simulink model "autopilot_stateflow_sldv_P05_test"  (Simulink 8.8)
settings: Solver=FixedStepDiscrete  StartTime=0.0  StopTime=10.0  FixedStep=0.1  RelTol=1e-3  EnableMultiTasking=on
libraries: simulink x38, sldvlib x17
settings OptimizationCC: ExpressionDepthLimit=2147483647
settings DebuggingCC: SolverPrmCheckMsg=warning
settings GRTTargetCC: CombineOutputUpdateFcns=on  GRTInterface=off
settings ConfigComp: DVMode=PropertyProving  DVMaxProcessTime=30000  DVTestSuiteOptimization=CombinedObjectives (Nonlinear Extended)  DVDetectDeadLogic=on  DVDetectActiveLogic=on  DVDetectFloatOverflow=off  DVProvingStrategy=FindViolation

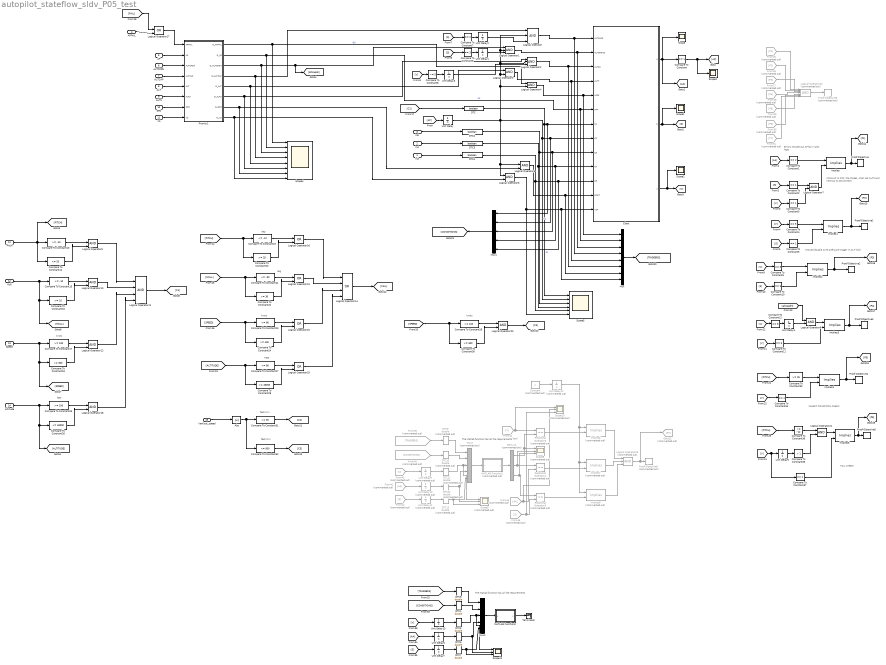
== system autopilot_stateflow_sldv_P05_test ==
  note: The Matlab function has all the requirements
  note: While AP is OFF, the Modes, shall set ALTS and
      | Vertical to Disconnect
  note: feet/min
  note: knots
  note: feet
  note: knots
  note: deg
  note: deg
  note: knots
  note: Feet
  note: feet/min
  note: FAIL CHECK
  note: INHIBIT CONDITION CHECK
  note: Missed disable ALTS software trigger in ALT hold
  note: Errors
      | Missed out AP fail in alts logic
  note: The Matlab function has all the requirements
  In3 : Inport
  In4 : Inport  Port=2
  In5 : Inport  Port=3
  APFAIL : Inport  Port=4
  AP : Inport  Port=5
  ALTCPDN : Inport  Port=6
  ALTCAP : Inport  Port=7
  ALT : Inport  Port=8
  ALTS : Inport  Port=9
  SPD : Inport  Port=10
  VS : Inport  Port=11
  Pitch : Inport  Port=12
  Speed : Inport  Port=13
  Altitude : Inport  Port=14
  Vertical_speed : Inport  Port=15
  Abs : Abs
  Chart : Stateflow chart  TreatAsAtomicUnit=on
  Compare To Constant{,2..3,5,34,37} (6 alike) : simulink/Logic and Bit Operations/Compare To Constant  relop===  const=1  OutDataTypeStr=boolean
  Compare To Constant1 : simulink/Logic and Bit Operations/Compare To Constant  relop===  const=2  OutDataTypeStr=boolean
  Compare To Constant10 : simulink/Logic and Bit Operations/Compare To Constant  relop===  const=3  OutDataTypeStr=boolean
  Compare To Constant11 : simulink/Logic and Bit Operations/Compare To Constant  relop===  const=5  OutDataTypeStr=boolean
  Compare To Constant12 : simulink/Logic and Bit Operations/Compare To Constant  relop===  const=6  OutDataTypeStr=boolean
  Compare To Constant13 : simulink/Logic and Bit Operations/Compare To Constant  relop=>=  const=-10  OutDataTypeStr=boolean
  Compare To Constant14 : simulink/Logic and Bit Operations/Compare To Constant  relop=<=  const=20  OutDataTypeStr=boolean
  Compare To Constant15 : simulink/Logic and Bit Operations/Compare To Constant  relop=>=  const=-10  OutDataTypeStr=boolean
  Compare To Constant16 : simulink/Logic and Bit Operations/Compare To Constant  relop=<=  const=10  OutDataTypeStr=boolean
  Compare To Constant17 : simulink/Logic and Bit Operations/Compare To Constant  relop=>=  const=100  OutDataTypeStr=boolean
  Compare To Constant18 : simulink/Logic and Bit Operations/Compare To Constant  relop=<=  const=300  OutDataTypeStr=boolean
  Compare To Constant19 : simulink/Logic and Bit Operations/Compare To Constant  relop=<=  const=-12  OutDataTypeStr=boolean
  Compare To Constant20 : simulink/Logic and Bit Operations/Compare To Constant  relop=>=  const=25  OutDataTypeStr=boolean
  Compare To Constant21 : simulink/Logic and Bit Operations/Compare To Constant  relop=<=  const=-30  OutDataTypeStr=boolean
  Compare To Constant22 : simulink/Logic and Bit Operations/Compare To Constant  relop=>=  const=30  OutDataTypeStr=boolean
  Compare To Constant23 : simulink/Logic and Bit Operations/Compare To Constant  relop=<=  const=80  OutDataTypeStr=boolean
  Compare To Constant24 : simulink/Logic and Bit Operations/Compare To Constant  relop=>=  const=400  OutDataTypeStr=boolean
  Compare To Constant25 : simulink/Logic and Bit Operations/Compare To Constant  relop=>=  const=100  OutDataTypeStr=boolean
  Compare To Constant26 : simulink/Logic and Bit Operations/Compare To Constant  relop=<=  const=40000  OutDataTypeStr=boolean
  Compare To Constant27 : simulink/Logic and Bit Operations/Compare To Constant  relop=<=  const=80  OutDataTypeStr=boolean
  Compare To Constant28 : simulink/Logic and Bit Operations/Compare To Constant  relop=>=  const=45000  OutDataTypeStr=boolean
  Compare To Constant29 : simulink/Logic and Bit Operations/Compare To Constant  relop=>=  const=120  OutDataTypeStr=boolean
  Compare To Constant30 : simulink/Logic and Bit Operations/Compare To Constant  relop=<=  const=300  OutDataTypeStr=boolean
  Compare To Constant31 : simulink/Logic and Bit Operations/Compare To Constant  relop=>=  const=50  OutDataTypeStr=boolean
  Compare To Constant32 : simulink/Logic and Bit Operations/Compare To Constant  relop=<=  const=500  OutDataTypeStr=boolean
  Compare To Constant33 : simulink/Logic and Bit Operations/Compare To Constant  relop=>=  const=25  OutDataTypeStr=boolean
  Compare To Constant35 : simulink/Logic and Bit Operations/Compare To Constant  relop=>  const=1  OutDataTypeStr=boolean
  Compare To Constant36 : simulink/Logic and Bit Operations/Compare To Constant  relop=<=  const=-12  OutDataTypeStr=boolean
  Compare To Constant4 : simulink/Logic and Bit Operations/Compare To Constant  relop===  const=5  OutDataTypeStr=boolean
  Compare To Constant6 : simulink/Logic and Bit Operations/Compare To Constant  relop===  const=3  OutDataTypeStr=boolean
  Compare To Constant7 : simulink/Logic and Bit Operations/Compare To Constant  relop===  const=2  OutDataTypeStr=boolean
  Compare To Constant8 : simulink/Logic and Bit Operations/Compare To Constant  relop=~=  const=5  OutDataTypeStr=boolean
  Compare To Constant9 : simulink/Logic and Bit Operations/Compare To Constant  relop===  const=6  OutDataTypeStr=boolean
  Constant : Constant  Commented=on
  DTC{,2..4} (4 alike) : DataTypeConversion  OutDataTypeStr=boolean
  DTC{1,5..8} (5 alike) : DataTypeConversion  OutDataTypeStr=double
  DTC{9..13} (5 alike) : DataTypeConversion  Commented=on  OutDataTypeStr=double
  Demux1 : Demux  Commented=on  Outputs=3
  From25 : From  Commented=on  GotoTag=P1
  From26 : From  Commented=on  GotoTag=P2
  From27 : From  Commented=on  GotoTag=P3
  From28 : From  Commented=on  GotoTag=P4
  From29 : From  Commented=on  GotoTag=P5
  From30 : From  Commented=on  GotoTag=P6
  From31 : From  Commented=on  GotoTag=P7
  From39 : From  Commented=on  GotoTag=TRIGGERS
  From40 : From  Commented=on  GotoTag=CONDITIONS
  From41 : From  Commented=on  GotoTag=AA
  From42 : From  Commented=on  GotoTag=S
  From43 : From  Commented=on  GotoTag=V
  From44 : From  Commented=on  GotoTag=V
  From45 : From  Commented=on  GotoTag=AA
  From46 : From  Commented=on  GotoTag=S
  Goto22 : Goto  Commented=on  GotoTag=P7
  Implies{,1..5} (6 alike) : sldvlib/Verification Utilities/Implies
  Implies6 : sldvlib/Verification Utilities/Implies  Commented=on
  Implies7 : sldvlib/Verification Utilities/Implies  Commented=on
  Implies8 : sldvlib/Verification Utilities/Implies  Commented=on
  Logical Operator : Logic  Inputs=3  IconShape=distinctive  AllPortsSameDT=off  OutDataTypeStr=boolean
  Logical Operator1 : Logic  Inputs=3  IconShape=distinctive  AllPortsSameDT=off  OutDataTypeStr=boolean
  Logical Operator{3..6,9..10,12,18,20} (9 alike) : Logic  IconShape=distinctive  AllPortsSameDT=off  OutDataTypeStr=boolean
  Logical Operator11 : Logic  Inputs=4  IconShape=distinctive  AllPortsSameDT=off  OutDataTypeStr=boolean
  Logical Operator{13,15..17,19} (5 alike) : Logic  Operator=OR  IconShape=distinctive  AllPortsSameDT=off  OutDataTypeStr=boolean
  Logical Operator14 : Logic  Operator=OR  Inputs=4  IconShape=distinctive  AllPortsSameDT=off  OutDataTypeStr=boolean
  Logical Operator2 : Logic  Inputs=3  IconShape=distinctive  AllPortsSameDT=off  OutDataTypeStr=boolean
  Logical Operator21 : Logic  AllPortsSameDT=off  OutDataTypeStr=boolean
  Logical Operator22 : Logic  Commented=on  Inputs=7  IconShape=distinctive  AllPortsSameDT=off  OutDataTypeStr=boolean
  Logical Operator23 : Logic  Commented=on  Inputs=3  IconShape=distinctive  AllPortsSameDT=off  OutDataTypeStr=boolean
  Logical Operator7 : Logic  AllPortsSameDT=off  OutDataTypeStr=boolean
  Logical Operator8 : Logic  AllPortsSameDT=off  OutDataTypeStr=boolean
  MATLAB Function1 : MATLAB Function  Commented=on  TreatAsAtomicUnit=on
  MATLAB Function2 : MATLAB Function  TreatAsAtomicUnit=on
  Mux : Mux  Inputs=8
  Mux1 : Mux  Inputs=5
  Mux2 : Mux  Inputs=5
  Mux3 : Mux  Commented=on  Inputs=5
  Priority1 : Subsystem
  Proof Objective{,1..5} (6 alike) : sldvlib/Objectives and Constraints/Proof Objective  enabled=off  customAVTBlockType=Proof Objective  intervals=true  dispValues=on  outEnabled=off  enableStopSim=off
      settings: AttributesFormatString=%<intervals>
  Proof Objective6 : sldvlib/Objectives and Constraints/Proof Objective  Commented=on  enabled=on  customAVTBlockType=Proof Objective  intervals=true  dispValues=on  outEnabled=off  enableStopSim=off
      settings: AttributesFormatString=%<intervals>
  Proof Objective8 : sldvlib/Objectives and Constraints/Proof Objective  Commented=on  enabled=off  customAVTBlockType=Proof Objective  intervals=true  dispValues=on  outEnabled=off  enableStopSim=off
      settings: AttributesFormatString=%<intervals>
  Relational Operator3 : RelationalOperator  Commented=on  Operator===  OutDataTypeStr=boolean  RndMeth=Simplest
  Relational Operator4 : RelationalOperator  Commented=on  Operator===  OutDataTypeStr=boolean  RndMeth=Simplest
  Relational Operator5 : RelationalOperator  Commented=on  Operator===  OutDataTypeStr=boolean  RndMeth=Simplest
  Roll : InportShadow  Port=12
  Scope{,1..3} (4 alike) : Scope
  Scope10 : Scope  Commented=on  NumInputPorts=3
  Scope11 : Scope  NumInputPorts=3
  Scope4 : Scope  NumInputPorts=8
  Scope5 : Scope  NumInputPorts=6
  Scope8 : Scope  Commented=on  NumInputPorts=3
  Scope9 : Scope  Commented=on  NumInputPorts=3
  Terminator : Terminator
  Unit Delay{,1..5} (6 alike) : UnitDelay  SampleTime=-1
  Unit Delay10 : UnitDelay  Commented=on  InitialCondition=2  SampleTime=-1
  Unit Delay11 : UnitDelay  Commented=on  InitialCondition=1  SampleTime=-1
  Unit Delay12 : UnitDelay  Commented=on  SampleTime=-1
  Unit Delay13 : UnitDelay  InitialCondition=1  SampleTime=-1
  Unit Delay6 : UnitDelay  InitialCondition=2  SampleTime=-1
  Unit Delay7 : UnitDelay  InitialCondition=1  SampleTime=-1
  Unit Delay9 : UnitDelay  Commented=on  InitialCondition=1  SampleTime=-1
  wires:
  Priority1/2(O_AP) -> Mux/2, Chart/6(APT), Scope4/2  "ap"
  [C1] -> DTC/1
  In5/1 -> DTC2/1
  In4/1 -> DTC3/1
  In3/1 -> DTC4/1
  DTC/1 -> Scope5/1, Mux1/1, Chart/7(C1)  "C1"
  DTC2/1 -> Scope5/3, Mux1/3, Chart/9(C3)
  DTC3/1 -> Scope5/4, Mux1/4, Chart/10(C4)
  DTC4/1 -> Scope5/5, Mux1/5, Chart/11(C5)
  Compare To Constant/1 -> Scope3/1, [AP]
  Chart/1(A) -> [AA], Compare To Constant/1, Scope/1
  [AP] -> Unit Delay/1
  Chart/2(S) -> Scope1/1, [S]
  Chart/3(V) -> Scope2/1, [V]
  Unit Delay/1 -> Scope5/2, Mux1/2, Chart/8(C2), Logical Operator6/1, Logical Operator5/1, Logical Operator3/2, Logical Operator/2, Logical Operator1/2, Logical Operator2/2, Logical Operator4/2  "C2"
  Logical Operator/1 -> Mux/4, Chart/1(ALTCAPS)
  Priority1/4(O_ALTCAP) -> Logical Operator/1, Scope4/4
  Logical Operator1/1 -> Mux/3, Chart/2(ALTCPDNS)
  Priority1/3(O_ALTCPDN) -> [altcapdn], Logical Operator1/1, Scope4/3
  Logical Operator2/1 -> Mux/6, Chart/3(ALTSS)
  Priority1/6(O_ALTS) -> Logical Operator2/1, Scope4/6
  Logical Operator3/1 -> Mux/5, Chart/4(ALTT)
  Priority1/5(O_ALT) -> Logical Operator3/1, Scope4/5
  Logical Operator4/1 -> Mux/1, Chart/5(APFS)
  Priority1/1(O_APFAIL) -> Logical Operator4/1, Scope4/1  "fail"
  Priority1/7(O_SPD) -> Logical Operator5/2, Scope4/7
  Logical Operator5/1 -> Mux/7, Chart/12(SPDT)
  Logical Operator6/1 -> Scope5/6, Mux/8, Chart/13(VST)
  Priority1/8(O_VS) -> Logical Operator6/2, Scope4/8
  ALT/1 -> Priority1/5(ALT)
  AP/1 -> Priority1/2(AP)
  ALTCAP/1 -> Priority1/4(ALTCAP)
  ALTS/1 -> Priority1/6(ALTS)
  SPD/1 -> Priority1/7(SPD)
  VS/1 -> Priority1/8(VS)
  ALTCPDN/1 -> Priority1/3(ALTCPDN)
  Unit Delay1/1 -> Logical Operator1/3
  [S] -> Compare To Constant6/1
  Compare To Constant6/1 -> Unit Delay1/1
  [S] -> Compare To Constant7/1
  Compare To Constant7/1 -> Unit Delay2/1
  Unit Delay2/1 -> Logical Operator/3
  [V] -> Compare To Constant8/1
  Compare To Constant8/1 -> Unit Delay3/1
  Unit Delay3/1 -> Logical Operator2/3
  Pitch/1 -> [PITCH], Compare To Constant14/1, Compare To Constant13/1
  Compare To Constant13/1 -> Logical Operator9/1
  Compare To Constant14/1 -> Logical Operator9/2
  Roll/1 -> Compare To Constant15/1, [ROLL], Compare To Constant16/1
  Compare To Constant15/1 -> Logical Operator10/1
  Compare To Constant16/1 -> Logical Operator10/2
  Speed/1 -> [SPEED], Compare To Constant18/1, Compare To Constant17/1
  Compare To Constant17/1 -> Logical Operator12/1
  Compare To Constant18/1 -> Logical Operator12/2
  Logical Operator9/1 -> Logical Operator11/1
  Logical Operator10/1 -> Logical Operator11/2
  Logical Operator12/1 -> Logical Operator11/3
  Logical Operator11/1 -> [C1]
  [PITCH] -> Compare To Constant19/1, Compare To Constant20/1
  Compare To Constant19/1 -> Logical Operator16/1
  Compare To Constant20/1 -> Logical Operator16/2
  [ROLL] -> Compare To Constant22/1, Compare To Constant21/1
  Compare To Constant21/1 -> Logical Operator13/1
  Compare To Constant22/1 -> Logical Operator13/2
  [SPEED] -> Compare To Constant23/1, Compare To Constant24/1
  Compare To Constant23/1 -> Logical Operator15/1
  Compare To Constant24/1 -> Logical Operator15/2
  Logical Operator16/1 -> Logical Operator14/1
  Logical Operator13/1 -> Logical Operator14/2
  Logical Operator15/1 -> Logical Operator14/3
  Logical Operator14/1 -> [FAIL]
  APFAIL/1 -> Logical Operator17/2
  [FAIL] -> Logical Operator17/1
  Logical Operator17/1 -> Priority1/1(APFAIL)
  Altitude/1 -> Compare To Constant25/1, Compare To Constant26/1, [ALTITUDE]
  Compare To Constant25/1 -> Logical Operator18/1
  Compare To Constant26/1 -> Logical Operator18/2
  Logical Operator18/1 -> Logical Operator11/4
  [ALTITUDE] -> Compare To Constant28/1, Compare To Constant27/1
  Compare To Constant27/1 -> Logical Operator19/1
  Compare To Constant28/1 -> Logical Operator19/2
  Logical Operator19/1 -> Logical Operator14/4
  [SPEED] -> Compare To Constant30/1, Compare To Constant29/1
  Compare To Constant29/1 -> Logical Operator20/1
  Compare To Constant30/1 -> Logical Operator20/2
  Logical Operator20/1 -> [C3]
  Vertical_speed/1 -> Abs/1
  Abs/1 -> Compare To Constant32/1, Compare To Constant31/1
  Compare To Constant31/1 -> [C4]
  Compare To Constant32/1 -> [C5]
  Compare To Constant1/1 -> Implies/1
  [AA] -> Compare To Constant1/1
  [S] -> Compare To Constant2/1
  Compare To Constant2/1 -> Logical Operator7/1
  [V] -> Compare To Constant3/1
  Compare To Constant3/1 -> Logical Operator7/2
  Logical Operator7/1 -> Implies/2
  Implies/1 -> [P1], Proof Objective/1
  [V] -> Compare To Constant4/1
  Compare To Constant4/1 -> Implies1/1
  [S] -> Compare To Constant5/1
  Compare To Constant5/1 -> Implies1/2
  Implies1/1 -> [P2], Proof Objective1/1
  [V] -> Compare To Constant9/1
  Compare To Constant9/1 -> Implies2/1
  [S] -> Compare To Constant10/1
  Compare To Constant10/1 -> Implies2/2
  Implies2/1 -> [P3], Proof Objective2/1
  [V] -> Compare To Constant12/1
  Compare To Constant12/1 -> Unit Delay4/1
  [V] -> Compare To Constant11/1
  Implies3/1 -> [P4], Proof Objective3/1
  Unit Delay4/1 -> Logical Operator8/2
  Logical Operator8/1 -> Implies3/1
  [altcapdn] -> Logical Operator8/1
  Compare To Constant11/1 -> Implies3/2
  [PITCH] -> Compare To Constant33/1
  Compare To Constant33/1 -> Implies4/1
  [V] -> Compare To Constant34/1
  Compare To Constant34/1 -> Implies4/2
  Implies4/1 -> [P5], Proof Objective4/1
  [V] -> Compare To Constant37/1, Unit Delay5/1
  [PITCH] -> Compare To Constant36/1
  Unit Delay5/1 -> Compare To Constant35/1
  Compare To Constant35/1 -> Logical Operator21/2
  Compare To Constant36/1 -> Logical Operator21/1
  Logical Operator21/1 -> Implies5/1
  Compare To Constant37/1 -> Implies5/2
  Implies5/1 -> [P6], Proof Objective5/1
  From28/1 -> Logical Operator22/4
  From27/1 -> Logical Operator22/3
  From29/1 -> Logical Operator22/5
  From26/1 -> Logical Operator22/2
  From30/1 -> Logical Operator22/6
  From25/1 -> Logical Operator22/1
  Logical Operator22/1 -> Proof Objective6/1
  Mux/1 -> [TRIGGERS]
  Mux1/1 -> [CONDITIONS]
  From40/1 -> DTC10/1
  From39/1 -> DTC9/1
  From43/1 -> Unit Delay9/1
  From41/1 -> Unit Delay10/1
  From42/1 -> Unit Delay11/1
  Mux3/1 -> MATLAB Function1/1(u)
  Unit Delay9/1 -> DTC11/1
  Unit Delay10/1 -> DTC12/1
  Unit Delay11/1 -> DTC13/1
  MATLAB Function1/1(y) -> Demux1/1
  From44/1 -> Scope10/1, Relational Operator3/1
  Demux1/1 -> Relational Operator3/2, Scope8/1
  Demux1/2 -> Relational Operator4/1, Scope8/2
  From45/1 -> Scope10/2, Relational Operator4/2
  Demux1/3 -> Relational Operator5/1, Scope8/3
  From46/1 -> Scope10/3, Relational Operator5/2
  DTC9/1 -> Mux3/1
  DTC10/1 -> Mux3/2
  DTC11/1 -> Mux3/3, Scope9/1
  DTC12/1 -> Mux3/4, Scope9/2
  DTC13/1 -> Mux3/5, Scope9/3
  Relational Operator3/1 -> Implies6/2
  Unit Delay12/1 -> Implies8/1, Implies7/1, Implies6/1
  Constant/1 -> Unit Delay12/1
  Relational Operator4/1 -> Implies7/2
  Relational Operator5/1 -> Implies8/2
  Implies7/1 -> Logical Operator23/2
  Implies6/1 -> Logical Operator23/1
  Implies8/1 -> Logical Operator23/3
  Logical Operator23/1 -> Goto22/1, Proof Objective8/1
  From31/1 -> Logical Operator22/7
  [CONDITIONS] -> DTC1/1
  [TRIGGERS] -> DTC8/1
  [V] -> Unit Delay13/1
  [AA] -> Unit Delay6/1
  [S] -> Unit Delay7/1
  Mux2/1 -> MATLAB Function2/1(u)
  Unit Delay13/1 -> DTC5/1
  Unit Delay6/1 -> DTC6/1
  Unit Delay7/1 -> DTC7/1
  DTC8/1 -> Mux2/1
  DTC1/1 -> Mux2/2
  DTC5/1 -> Scope11/1, Mux2/3
  DTC6/1 -> Scope11/2, Mux2/4
  DTC7/1 -> Scope11/3, Mux2/5
  MATLAB Function2/1(y) -> Terminator/1

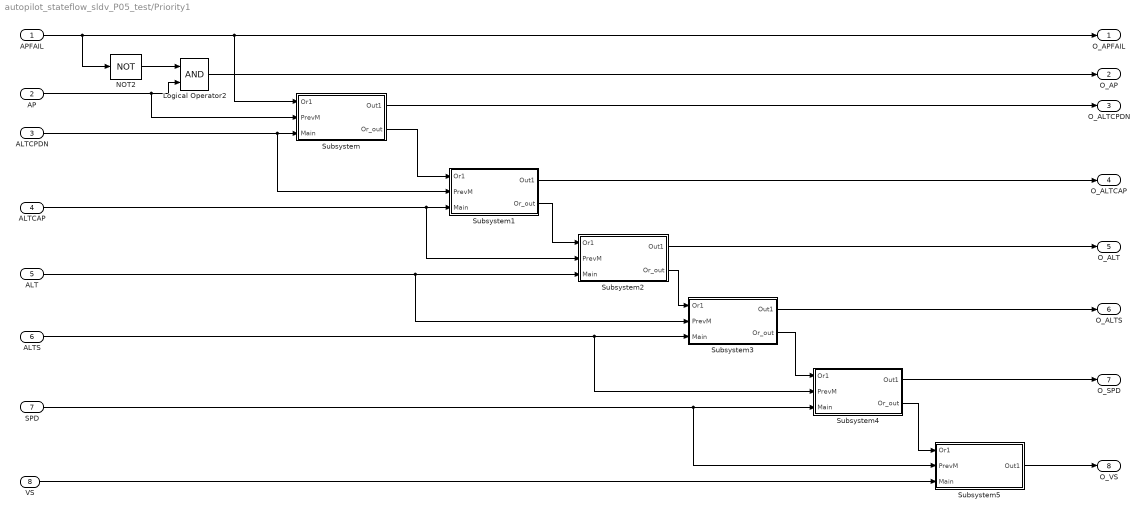
== system autopilot_stateflow_sldv_P05_test/Priority1 ==
  APFAIL : Inport
  AP : Inport  Port=2
  ALTCPDN : Inport  Port=3
  ALTCAP : Inport  Port=4
  ALT : Inport  Port=5
  ALTS : Inport  Port=6
  SPD : Inport  Port=7
  VS : Inport  Port=8
  Logical Operator2 : Logic  AllPortsSameDT=off  OutDataTypeStr=boolean
  NOT2 : Logic  Operator=NOT  AllPortsSameDT=off  OutDataTypeStr=boolean
  Subsystem : Subsystem
  Subsystem1 : Subsystem
  Subsystem2 : Subsystem
  Subsystem3 : Subsystem
  Subsystem4 : Subsystem
  Subsystem5 : Subsystem
  O_APFAIL : Outport
  O_AP : Outport  Port=2
  O_ALTCPDN : Outport  Port=3
  O_ALTCAP : Outport  Port=4
  O_ALT : Outport  Port=5
  O_ALTS : Outport  Port=6
  O_SPD : Outport  Port=7
  O_VS : Outport  Port=8
  wires:
  AP/1 -> Subsystem/2(PrevM), Logical Operator2/2
  APFAIL/1 -> Subsystem/1(Or1), O_APFAIL/1, NOT2/1
  NOT2/1 -> Logical Operator2/1
  Logical Operator2/1 -> O_AP/1
  ALTCPDN/1 -> Subsystem1/2(PrevM), Subsystem/3(Main)
  Subsystem/2(Or_out) -> Subsystem1/1(Or1)
  ALTCAP/1 -> Subsystem2/2(PrevM), Subsystem1/3(Main)
  Subsystem/1(Out1) -> O_ALTCPDN/1
  Subsystem1/1(Out1) -> O_ALTCAP/1
  Subsystem1/2(Or_out) -> Subsystem2/1(Or1)
  ALT/1 -> Subsystem3/2(PrevM), Subsystem2/3(Main)
  Subsystem2/1(Out1) -> O_ALT/1
  Subsystem2/2(Or_out) -> Subsystem3/1(Or1)
  ALTS/1 -> Subsystem4/2(PrevM), Subsystem3/3(Main)
  Subsystem3/1(Out1) -> O_ALTS/1
  Subsystem3/2(Or_out) -> Subsystem4/1(Or1)
  SPD/1 -> Subsystem5/2(PrevM), Subsystem4/3(Main)
  Subsystem4/1(Out1) -> O_SPD/1
  Subsystem4/2(Or_out) -> Subsystem5/1(Or1)
  VS/1 -> Subsystem5/3(Main)
  Subsystem5/1(Out1) -> O_VS/1

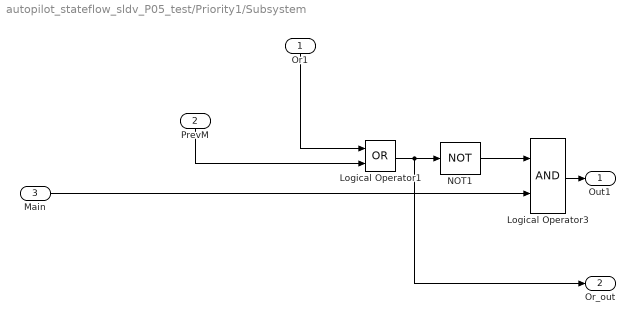
== system autopilot_stateflow_sldv_P05_test/Priority1/Subsystem ==
  Or1 : Inport
  PrevM : Inport  Port=2
  Main : Inport  Port=3
  Logical Operator1 : Logic  Operator=OR  AllPortsSameDT=off  OutDataTypeStr=boolean
  Logical Operator3 : Logic  AllPortsSameDT=off  OutDataTypeStr=boolean
  NOT1 : Logic  Operator=NOT  AllPortsSameDT=off  OutDataTypeStr=boolean
  Out1 : Outport
  Or_out : Outport  Port=2
  wires:
  Main/1 -> Logical Operator3/2
  Logical Operator1/1 -> Or_out/1, NOT1/1
  NOT1/1 -> Logical Operator3/1
  Or1/1 -> Logical Operator1/1
  Logical Operator3/1 -> Out1/1
  PrevM/1 -> Logical Operator1/2

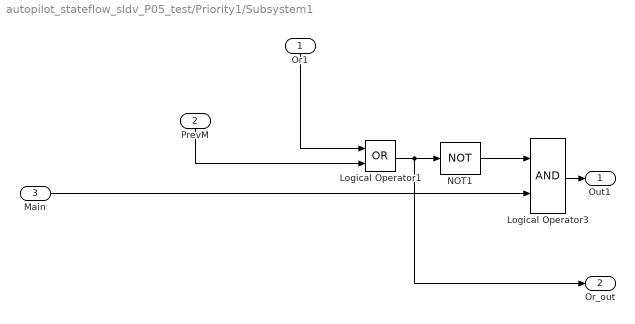
== system autopilot_stateflow_sldv_P05_test/Priority1/Subsystem1 ==
  Or1 : Inport
  PrevM : Inport  Port=2
  Main : Inport  Port=3
  Logical Operator1 : Logic  Operator=OR  AllPortsSameDT=off  OutDataTypeStr=boolean
  Logical Operator3 : Logic  AllPortsSameDT=off  OutDataTypeStr=boolean
  NOT1 : Logic  Operator=NOT  AllPortsSameDT=off  OutDataTypeStr=boolean
  Out1 : Outport
  Or_out : Outport  Port=2
  wires:
  PrevM/1 -> Logical Operator1/2
  Logical Operator3/1 -> Out1/1
  Or1/1 -> Logical Operator1/1
  NOT1/1 -> Logical Operator3/1
  Logical Operator1/1 -> NOT1/1, Or_out/1
  Main/1 -> Logical Operator3/2

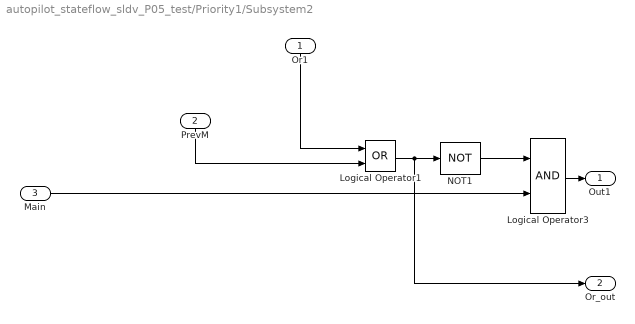
== system autopilot_stateflow_sldv_P05_test/Priority1/Subsystem2 ==
  Or1 : Inport
  PrevM : Inport  Port=2
  Main : Inport  Port=3
  Logical Operator1 : Logic  Operator=OR  AllPortsSameDT=off  OutDataTypeStr=boolean
  Logical Operator3 : Logic  AllPortsSameDT=off  OutDataTypeStr=boolean
  NOT1 : Logic  Operator=NOT  AllPortsSameDT=off  OutDataTypeStr=boolean
  Out1 : Outport
  Or_out : Outport  Port=2
  wires:
  Main/1 -> Logical Operator3/2
  Logical Operator1/1 -> Or_out/1, NOT1/1
  NOT1/1 -> Logical Operator3/1
  Or1/1 -> Logical Operator1/1
  Logical Operator3/1 -> Out1/1
  PrevM/1 -> Logical Operator1/2

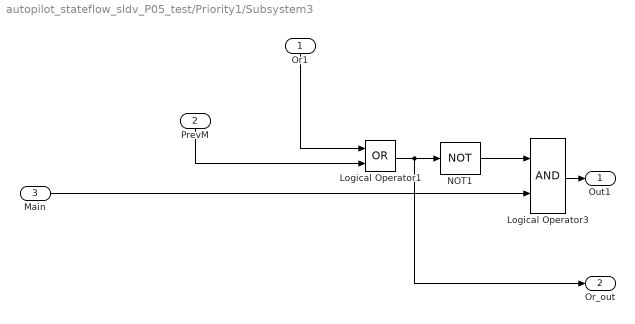
== system autopilot_stateflow_sldv_P05_test/Priority1/Subsystem3 ==
  Or1 : Inport
  PrevM : Inport  Port=2
  Main : Inport  Port=3
  Logical Operator1 : Logic  Operator=OR  AllPortsSameDT=off  OutDataTypeStr=boolean
  Logical Operator3 : Logic  AllPortsSameDT=off  OutDataTypeStr=boolean
  NOT1 : Logic  Operator=NOT  AllPortsSameDT=off  OutDataTypeStr=boolean
  Out1 : Outport
  Or_out : Outport  Port=2
  wires:
  PrevM/1 -> Logical Operator1/2
  Logical Operator3/1 -> Out1/1
  Or1/1 -> Logical Operator1/1
  NOT1/1 -> Logical Operator3/1
  Logical Operator1/1 -> NOT1/1, Or_out/1
  Main/1 -> Logical Operator3/2

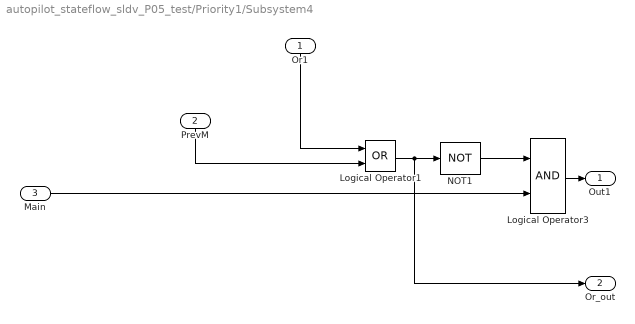
== system autopilot_stateflow_sldv_P05_test/Priority1/Subsystem4 ==
  Or1 : Inport
  PrevM : Inport  Port=2
  Main : Inport  Port=3
  Logical Operator1 : Logic  Operator=OR  AllPortsSameDT=off  OutDataTypeStr=boolean
  Logical Operator3 : Logic  AllPortsSameDT=off  OutDataTypeStr=boolean
  NOT1 : Logic  Operator=NOT  AllPortsSameDT=off  OutDataTypeStr=boolean
  Out1 : Outport
  Or_out : Outport  Port=2
  wires:
  Main/1 -> Logical Operator3/2
  Logical Operator1/1 -> Or_out/1, NOT1/1
  NOT1/1 -> Logical Operator3/1
  Or1/1 -> Logical Operator1/1
  Logical Operator3/1 -> Out1/1
  PrevM/1 -> Logical Operator1/2

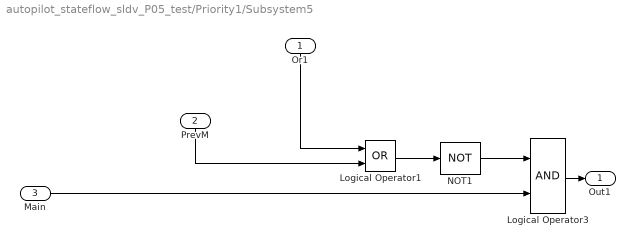
== system autopilot_stateflow_sldv_P05_test/Priority1/Subsystem5 ==
  Or1 : Inport
  PrevM : Inport  Port=2
  Main : Inport  Port=3
  Logical Operator1 : Logic  Operator=OR  AllPortsSameDT=off  OutDataTypeStr=boolean
  Logical Operator3 : Logic  AllPortsSameDT=off  OutDataTypeStr=boolean
  NOT1 : Logic  Operator=NOT  AllPortsSameDT=off  OutDataTypeStr=boolean
  Out1 : Outport
  wires:
  PrevM/1 -> Logical Operator1/2
  Logical Operator3/1 -> Out1/1
  Or1/1 -> Logical Operator1/1
  NOT1/1 -> Logical Operator3/1
  Logical Operator1/1 -> NOT1/1
  Main/1 -> Logical Operator3/2

== stateflow chart Chart ==
  state VERT [parallel]
    settings: executionOrder=1
    state DIS_01
      en: V = 1;
    state SPDH_03
      en: V = 3;
    state ALT_05
      en: V = 5;
    state PAH_02
      en: V = 2;
    state VS_04
      en: V = 4;
    state ALTSCAP_06
      en: V = 6;
    SPDH_03 -> DIS_01 [order 6] : [APFS & C2]
    (default) -> DIS_01
    SPDH_03 -> DIS_01 [order 1] : [APT & C2]
    SPDH_03 -> ALT_05 [order 4] : [ALTT & C5]
    DIS_01 -> PAH_02 : [APT & C1]
    PAH_02 -> SPDH_03 [order 2] : [SPDT & C3]
    ALT_05 -> DIS_01 [order 5] : [APFS & C2]
    ALT_05 -> SPDH_03 [order 2] : [SPDT & C3]
    ALT_05 -> DIS_01 [order 1] : [APT & C2]
    SPDH_03 -> PAH_02 [order 2] : [SPDT]
    VS_04 -> SPDH_03 [order 2] : [SPDT & C3]
    PAH_02 -> DIS_01 [order 6] : [APFS & C2]
    PAH_02 -> DIS_01 [order 1] : [APT & C2]
    ALTSCAP_06 -> DIS_01 [order 4] : [APFS & C2]
    ALTSCAP_06 -> DIS_01 [order 1] : [APT & C2]
    VS_04 -> DIS_01 [order 6] : [APFS & C2]
    VS_04 -> DIS_01 [order 1] : [APT & C2]
    SPDH_03 -> ALTSCAP_06 [order 5] : [ALTCAPS]
    SPDH_03 -> VS_04 [order 3] : [VST & C4]
    VS_04 -> ALT_05 [order 4] : [ALTT & C5]
    ALT_05 -> PAH_02 [order 4] : [ALTT]
    PAH_02 -> ALT_05 [order 4] : [ALTT & C5]
    ALTSCAP_06 -> ALT_05 [order 2] : [ALTT & C5]
    ALTSCAP_06 -> ALT_05 [order 3] : [ALTCPDNS]
    ALT_05 -> VS_04 [order 3] : [VST & C4]
    PAH_02 -> ALTSCAP_06 [order 5] : [ALTCAPS]
    PAH_02 -> VS_04 [order 3] : [VST & C4]
    VS_04 -> PAH_02 [order 3] : [VST]
    VS_04 -> ALTSCAP_06 [order 5] : [ALTCAPS]
  state AP [parallel]
    settings: executionOrder=2
    state ON_01
      en: A = 1;
    state OFF_02
      en: A = 2;
    OFF_02 -> ON_01 : [APT & C1]
    ON_01 -> OFF_02 [order 1] : [APT]
    ON_01 -> OFF_02 [order 2] : [APFS]
    (default) -> OFF_02
  state ALTSEL [parallel]
    settings: executionOrder=3
    state OFF_01
      en: S = 1;
    state CAP_03
      en: S = 3;
    state ARM_02
      en: S = 2;
    (default) -> OFF_01
    CAP_03 -> OFF_01 [order 4] : [APFS & C2]
    ARM_02 -> OFF_01 [order 3] : [ALTSS]
    CAP_03 -> OFF_01 [order 1] : [APT & C2]
    OFF_01 -> ARM_02 : [ALTSS]
    ARM_02 -> OFF_01 [order 2] : [APT & C2]
    ARM_02 -> OFF_01 [order 5] : [APFS & C2]
    ARM_02 -> OFF_01 [order 1] : [ALTT & C5]
    CAP_03 -> OFF_01 [order 3] : [ALTCPDNS]
    CAP_03 -> OFF_01 [order 2] : [ALTT & C5]
    ARM_02 -> CAP_03 [order 4] : [ALTCAPS]
  data: ALTCAPS input boolean; ALTCPDNS input boolean; ALTSS input boolean; ALTT input boolean; APFS input boolean; APT input boolean; C1 input boolean; C2 input boolean; C3 input boolean; C4 input boolean; C5 input boolean; SPDT input boolean; VST input boolean; A output uint32; S output uint32; V output uint32

== matlab function MATLAB Function2 ==
  data: u input double; y output double
function y = fcn(u)

nt = 8 ; nc = 5 ;
Tr = zeros(nt,1); C = zeros(nc,1);
for i = 1:nt; Tr(i) = u(i,1); end  % Assign triggers from input U
for i = 1:nc; C(i) = u(i+nt,1); end % Assign conditions from input U
V = u(14,1);
AP = u(15,1);
AS = u(16,1);
% Assign the trigger to one based on priority
% Add additonal conditions to enable triggers here
TRIG = 0;
if  Tr(1) == 1, TRIG = 1;  % APFAIL
elseif  Tr(2) == 1, TRIG = 2;  % AP
elseif  Tr(3) == 1, TRIG = 3;  % ALTCPDN
elseif  Tr(4) == 1, TRIG = 4;  % ALTCAP
elseif  Tr(5) == 1, TRIG = 5;  % ALT
elseif  Tr(6) == 1, TRIG = 6;  % ALTS
elseif  Tr(7) == 1, TRIG = 7;  % SPD
elseif  Tr(8) == 1, TRIG = 8;  % VS
end
% 1) While in State DIS AND Trigger AP occurs THEN transit to PAH if condition C1 is True
if  (V == 1) && (TRIG == 2) && (C(1) == 1) ; V = 2;
sldv.prove(V ~= 2,' 1) While in State DIS AND Trigger AP occurs THEN transit to PAH if condition C1 is True');
% 2) While in State PAH AND Trigger APFAIL occurs THEN transit to DIS if condition C2 is True
elseif  (V == 2) && (TRIG == 1) && (C(2) == 1) ; V = 1;
sldv.prove(V ~= 1,' 2) While in State PAH AND Trigger APFAIL occurs THEN transit to DIS if condition C2 is True');
% 3) While in State PAH AND Trigger AP occurs THEN transit to DIS if condition C2 is True
elseif  (V == 2) && (TRIG == 2) && (C(2) == 1) ; V = 1;
sldv.prove(V ~= 1,' 3) While in State PAH AND Trigger AP occurs THEN transit to DIS if condition C2 is True');
% 4) While in State PAH AND Trigger ALTCAP occurs THEN transit to ALTS_CAP if condition  [No Condition required] 
elseif  (V == 2) && (TRIG == 4)  ; V = 6;
sldv.prove(V ~= 6,' 4) While in State PAH AND Trigger ALTCAP occurs THEN transit to ALTS_CAP if condition  [No Condition required] ');
% 5) While in State PAH AND Trigger ALT occurs THEN transit to ALT_HOLD if condition C5 is True
elseif  (V == 2) && (TRIG == 5) && (C(5) == 1) ; V = 5;
sldv.prove(V ~= 5,' 5) While in State PAH AND Trigger ALT occurs THEN transit to ALT_HOLD if condition C5 is True');
% 6) While in State PAH AND Trigger SPD occurs THEN transit to SPD_HOLD if condition C3 is True
elseif  (V == 2) && (TRIG == 7) && (C(3) == 1) ; V = 3;
sldv.prove(V ~= 3,' 6) While in State PAH AND Trigger SPD occurs THEN transit to SPD_HOLD if condition C3 is True');
% 7) While in State PAH AND Trigger VS occurs THEN transit to VS if condition C4 is True
elseif  (V == 2) && (TRIG == 8) && (C(4) == 1) ; V = 4;
sldv.prove(V ~= 4,' 7) While in State PAH AND Trigger VS occurs THEN transit to VS if condition C4 is True');
% 8) While in State SPD_HOLD AND Trigger APFAIL occurs THEN transit to DIS if condition C2 is True
elseif  (V == 3) && (TRIG == 1) && (C(2) == 1) ; V = 1;
sldv.prove(V ~= 1,' 8) While in State SPD_HOLD AND Trigger APFAIL occurs THEN transit to DIS if condition C2 is True');
% 9) While in State SPD_HOLD AND Trigger AP occurs THEN transit to DIS if condition C2 is True
elseif  (V == 3) && (TRIG == 2) && (C(2) == 1) ; V = 1;
sldv.prove(V ~= 1,' 9) While in State SPD_HOLD AND Trigger AP occurs THEN transit to DIS if condition C2 is True');
% 10) While in State SPD_HOLD AND Trigger ALTCAP occurs THEN transit to ALTS_CAP if condition  [No Condition required] 
elseif  (V == 3) && (TRIG == 4)  ; V = 6;
sldv.prove(V ~= 6,' 10) While in State SPD_HOLD AND Trigger ALTCAP occurs THEN transit to ALTS_CAP if condition  [No Condition required] ');
% 11) While in State SPD_HOLD AND Trigger ALT occurs THEN transit to ALT_HOLD if condition C5 is True
elseif  (V == 3) && (TRIG == 5) && (C(5) == 1) ; V = 5;
sldv.prove(V ~= 5,' 11) While in State SPD_HOLD AND Trigger ALT occurs THEN transit to ALT_HOLD if condition C5 is True');
% 12) While in State SPD_HOLD AND Trigger SPD occurs THEN transit to PAH if condition  [No Condition required] 
elseif  (V == 3) && (TRIG == 7)  ; V = 2;
sldv.prove(V ~= 2,' 12) While in State SPD_HOLD AND Trigger SPD occurs THEN transit to PAH if condition  [No Condition required] ');
% 13) While in State SPD_HOLD AND Trigger VS occurs THEN transit to VS if condition C4 is True
elseif  (V == 3) && (TRIG == 8) && (C(4) == 1) ; V = 4;
sldv.prove(V ~= 4,' 13) While in State SPD_HOLD AND Trigger VS occurs THEN transit to VS if condition C4 is True');
% 14) While in State VS AND Trigger APFAIL occurs THEN transit to DIS if condition C2 is True
elseif  (V == 4) && (TRIG == 1) && (C(2) == 1) ; V = 1;
sldv.prove(V ~= 1,' 14) While in State VS AND Trigger APFAIL occurs THEN transit to DIS if condition C2 is True');
% 15) While in State VS AND Trigger AP occurs THEN transit to DIS if condition C2 is True
elseif  (V == 4) && (TRIG == 2) && (C(2) == 1) ; V = 1;
sldv.prove(V ~= 1,' 15) While in State VS AND Trigger AP occurs THEN transit to DIS if condition C2 is True');
% 16) While in State VS AND Trigger ALTCAP occurs THEN transit to ALTS_CAP if condition  [No Condition required] 
elseif  (V == 4) && (TRIG == 4)  ; V = 6;
sldv.prove(V ~= 6,' 16) While in State VS AND Trigger ALTCAP occurs THEN transit to ALTS_CAP if condition  [No Condition required] ');
% 17) While in State VS AND Trigger ALT occurs THEN transit to ALT_HOLD if condition C5 is True
elseif  (V == 4) && (TRIG == 5) && (C(5) == 1) ; V = 5;
sldv.prove(V ~= 5,' 17) While in State VS AND Trigger ALT occurs THEN transit to ALT_HOLD if condition C5 is True');
% 18) While in State VS AND Trigger SPD occurs THEN transit to SPD_HOLD if condition C3 is True
elseif  (V == 4) && (TRIG == 7) && (C(3) == 1) ; V = 3;
sldv.prove(V ~= 3,' 18) While in State VS AND Trigger SPD occurs THEN transit to SPD_HOLD if condition C3 is True');
% 19) While in State VS AND Trigger VS occurs THEN transit to PAH if condition  [No Condition required] 
elseif  (V == 4) && (TRIG == 8)  ; V = 2;
sldv.prove(V ~= 2,' 19) While in State VS AND Trigger VS occurs THEN transit to PAH if condition  [No Condition required] ');
% 20) While in State ALT_HOLD AND Trigger APFAIL occurs THEN transit to DIS if condition C2 is True
elseif  (V == 5) && (TRIG == 1) && (C(2) == 1) ; V = 1;
sldv.prove(V ~= 1,' 20) While in State ALT_HOLD AND Trigger APFAIL occurs THEN transit to DIS if condition C2 is True');
% 21) While in State ALT_HOLD AND Trigger AP occurs THEN transit to DIS if condition C2 is True
elseif  (V == 5) && (TRIG == 2) && (C(2) == 1) ; V = 1;
sldv.prove(V ~= 1,' 21) While in State ALT_HOLD AND Trigger AP occurs THEN transit to DIS if condition C2 is True');
% 22) While in State ALT_HOLD AND Trigger ALT occurs THEN transit to PAH if condition  [No Condition required] 
elseif  (V == 5) && (TRIG == 5)  ; V = 2;
sldv.prove(V ~= 2,' 22) While in State ALT_HOLD AND Trigger ALT occurs THEN transit to PAH if condition  [No Condition required] ');
% 23) While in State ALT_HOLD AND Trigger SPD occurs THEN transit to SPD_HOLD if condition C3 is True
elseif  (V == 5) && (TRIG == 7) && (C(3) == 1) ; V = 3;
sldv.prove(V ~= 3,' 23) While in State ALT_HOLD AND Trigger SPD occurs THEN transit to SPD_HOLD if condition C3 is True');
% 24) While in State ALT_HOLD AND Trigger VS occurs THEN transit to VS if condition C4 is True
elseif  (V == 5) && (TRIG == 8) && (C(4) == 1) ; V = 4;
sldv.prove(V ~= 4,' 24) While in State ALT_HOLD AND Trigger VS occurs THEN transit to VS if condition C4 is True');
% 25) While in State ALTS_CAP AND Trigger APFAIL occurs THEN transit to DIS if condition C2 is True
elseif  (V == 6) && (TRIG == 1) && (C(2) == 1) ; V = 1;
sldv.prove(V ~= 1,' 25) While in State ALTS_CAP AND Trigger APFAIL occurs THEN transit to DIS if condition C2 is True');
% 26) While in State ALTS_CAP AND Trigger AP occurs THEN transit to DIS if condition C2 is True
elseif  (V == 6) && (TRIG == 2) && (C(2) == 1) ; V = 1;
sldv.prove(V ~= 1,' 26) While in State ALTS_CAP AND Trigger AP occurs THEN transit to DIS if condition C2 is True');
% 27) While in State ALTS_CAP AND Trigger ALTCPDN occurs THEN transit to ALT_HOLD if condition  [No Condition required] 
elseif  (V == 6) && (TRIG == 3)  ; V = 5;
sldv.prove(V ~= 5,' 27) While in State ALTS_CAP AND Trigger ALTCPDN occurs THEN transit to ALT_HOLD if condition  [No Condition required] ');
% 28) While in State ALTS_CAP AND Trigger ALT occurs THEN transit to ALT_HOLD if condition C5 is True
elseif  (V == 6) && (TRIG == 5) && (C(5) == 1) ; V = 5;
sldv.prove(V ~= 5,' 28) While in State ALTS_CAP AND Trigger ALT occurs THEN transit to ALT_HOLD if condition C5 is True');
end     
%   ================================================
  
% 29) While in State APON AND Trigger APFAIL occurs THEN transit to APOFF if condition  [No Condition required] 
if  (AP == 1) && (TRIG == 1)  ; AP = 2;
sldv.prove(AP ~= 2,' 29) While in State APON AND Trigger APFAIL occurs THEN transit to APOFF if condition  [No Condition required] ');
% 30) While in State APON AND Trigger AP occurs THEN transit to APOFF if condition  [No Condition required] 
elseif  (AP == 1) && (TRIG == 2)  ; AP = 2;
sldv.prove(AP ~= 2,' 30) While in State APON AND Trigger AP occurs THEN transit to APOFF if condition  [No Condition required] ');
% 31) While in State APOFF AND Trigger AP occurs THEN transit to APON if condition C1 is True
elseif  (AP == 2) && (TRIG == 2) && (C(1) == 1) ; AP = 1;
sldv.prove(AP ~= 1,' 31) While in State APOFF AND Trigger AP occurs THEN transit to APON if condition C1 is True');
end     
%   ================================================
  
% 32) While in State ALTSOFF AND Trigger ALTS occurs THEN transit to ALTSARM if condition  [No Condition required] 
if  (AS == 1) && (TRIG == 6)  ; AS = 2;
sldv.prove(AS ~= 2,' 32) While in State ALTSOFF AND Trigger ALTS occurs THEN transit to ALTSARM if condition  [No Condition required] ');
% 33) While in State ALTSARM AND Trigger APFAIL occurs THEN transit to ALTSOFF if condition C2 is True
elseif  (AS == 2) && (TRIG == 1) && (C(2) == 1) ; AS = 1;
sldv.prove(AS ~= 1,' 33) While in State ALTSARM AND Trigger APFAIL occurs THEN transit to ALTSOFF if condition C2 is True');
% 34) While in State ALTSARM AND Trigger AP occurs THEN transit to ALTSOFF if condition C2 is True
elseif  (AS == 2) && (TRIG == 2) && (C(2) == 1) ; AS = 1;
sldv.prove(AS ~= 1,' 34) While in State ALTSARM AND Trigger AP occurs THEN transit to ALTSOFF if condition C2 is True');
% 35) While in State ALTSARM AND Trigger ALTCAP occurs THEN transit to ALTSCAP if condition  [No Condition required] 
elseif  (AS == 2) && (TRIG == 4)  ; AS = 3;
sldv.prove(AS ~= 3,' 35) While in State ALTSARM AND Trigger ALTCAP occurs THEN transit to ALTSCAP if condition  [No Condition required] ');
% 36) While in State ALTSARM AND Trigger ALT occurs THEN transit to ALTSOFF if condition C5 is True
elseif  (AS == 2) && (TRIG == 5) && (C(5) == 1) ; AS = 1;
sldv.prove(AS ~= 1,' 36) While in State ALTSARM AND Trigger ALT occurs THEN transit to ALTSOFF if condition C5 is True');
% 37) While in State ALTSARM AND Trigger ALTS occurs THEN transit to ALTSOFF if condition  [No Condition required] 
elseif  (AS == 2) && (TRIG == 6)  ; AS = 1;
sldv.prove(AS ~= 1,' 37) While in State ALTSARM AND Trigger ALTS occurs THEN transit to ALTSOFF if condition  [No Condition required] ');
% 38) While in State ALTSCAP AND Trigger APFAIL occurs THEN transit to ALTSOFF if condition C2 is True
elseif  (AS == 3) && (TRIG == 1) && (C(2) == 1) ; AS = 1;
sldv.prove(AS ~= 1,' 38) While in State ALTSCAP AND Trigger APFAIL occurs THEN transit to ALTSOFF if condition C2 is True');
% 39) While in State ALTSCAP AND Trigger AP occurs THEN transit to ALTSOFF if condition C2 is True
elseif  (AS == 3) && (TRIG == 2) && (C(2) == 1) ; AS = 1;
sldv.prove(AS ~= 1,' 39) While in State ALTSCAP AND Trigger AP occurs THEN transit to ALTSOFF if condition C2 is True');
% 40) While in State ALTSCAP AND Trigger ALTCPDN occurs THEN transit to ALTSOFF if condition  [No Condition required] 
elseif  (AS == 3) && (TRIG == 3)  ; AS = 1;
sldv.prove(AS ~= 1,' 40) While in State ALTSCAP AND Trigger ALTCPDN occurs THEN transit to ALTSOFF if condition  [No Condition required] ');
% 41) While in State ALTSCAP AND Trigger ALT occurs THEN transit to ALTSOFF if condition C5 is True
elseif  (AS == 3) && (TRIG == 5) && (C(5) == 1) ; AS = 1;
sldv.prove(AS ~= 1,' 41) While in State ALTSCAP AND Trigger ALT occurs THEN transit to ALTSOFF if condition C5 is True');
end     
%   ================================================
  
% ============== Set the outputs ===========
y = zeros(3,1);
y(1) = V;
y(2) = AP;
y(3) = AS;

== matlab function MATLAB Function1 ==
  data: u input double; y output double
function y = fcn(u)

nt = 8 ; nc = 5 ;
Tr = zeros(nt,1); C = zeros(nc,1);
for i = 1:nt; Tr(i) = u(i,1); end  % Assign triggers from input U
for i = 1:nc; C(i) = u(i+nt,1); end % Assign conditions from input U
V = u(14,1);
AP = u(15,1);
AS = u(16,1);
% Assign the trigger to one based on priority
% Add additonal conditions to enable triggers here
TRIG = 0;
if  Tr(1) == 1, TRIG = 1;  % APFAIL
elseif  Tr(2) == 1, TRIG = 2;  % AP
elseif  Tr(3) == 1, TRIG = 3;  % ALTCPDN
elseif  Tr(4) == 1, TRIG = 4;  % ALTCAP
elseif  Tr(5) == 1, TRIG = 5;  % ALT
elseif  Tr(6) == 1, TRIG = 6;  % ALTS
elseif  Tr(7) == 1, TRIG = 7;  % SPD
elseif  Tr(8) == 1, TRIG = 8;  % VS
end
% 1) If in State DIS AND Trigger AP occurs THEN transit to PAH if condition C1 is True
if  (V == 1) && (TRIG == 2) && (C(1) == 1) ; V = 2;
% 2) If in State PAH AND Trigger APFAIL occurs THEN transit to DIS if condition C2 is True
elseif  (V == 2) && (TRIG == 1) && (C(2) == 1) ; V = 1;
% 3) If in State PAH AND Trigger AP occurs THEN transit to DIS if condition C2 is True
elseif  (V == 2) && (TRIG == 2) && (C(2) == 1) ; V = 1;
% 4) If in State PAH AND Trigger ALTCAP occurs THEN transit to ALTS_CAP if condition  [No Condition required] 
elseif  (V == 2) && (TRIG == 4)  ; V = 6;
% 5) If in State PAH AND Trigger ALT occurs THEN transit to ALT_HOLD if condition C5 is True
elseif  (V == 2) && (TRIG == 5) && (C(5) == 1) ; V = 5;
% 6) If in State PAH AND Trigger SPD occurs THEN transit to SPD_HOLD if condition C3 is True
elseif  (V == 2) && (TRIG == 7) && (C(3) == 1) ; V = 3;
% 7) If in State PAH AND Trigger VS occurs THEN transit to VS if condition C4 is True
elseif  (V == 2) && (TRIG == 8) && (C(4) == 1) ; V = 4;
% 8) If in State SPD_HOLD AND Trigger APFAIL occurs THEN transit to DIS if condition C2 is True
elseif  (V == 3) && (TRIG == 1) && (C(2) == 1) ; V = 1;
% 9) If in State SPD_HOLD AND Trigger AP occurs THEN transit to DIS if condition C2 is True
elseif  (V == 3) && (TRIG == 2) && (C(2) == 1) ; V = 1;
% 10) If in State SPD_HOLD AND Trigger ALTCAP occurs THEN transit to ALTS_CAP if condition  [No Condition required] 
elseif  (V == 3) && (TRIG == 4)  ; V = 6;
% 11) If in State SPD_HOLD AND Trigger ALT occurs THEN transit to ALT_HOLD if condition C5 is True
elseif  (V == 3) && (TRIG == 5) && (C(5) == 1) ; V = 5;
% 12) If in State SPD_HOLD AND Trigger SPD occurs THEN transit to PAH if condition  [No Condition required] 
elseif  (V == 3) && (TRIG == 7)  ; V = 2;
% 13) If in State SPD_HOLD AND Trigger VS occurs THEN transit to VS if condition C4 is True
elseif  (V == 3) && (TRIG == 8) && (C(4) == 1) ; V = 4;
% 14) If in State VS AND Trigger APFAIL occurs THEN transit to DIS if condition C2 is True
elseif  (V == 4) && (TRIG == 1) && (C(2) == 1) ; V = 1;
% 15) If in State VS AND Trigger AP occurs THEN transit to DIS if condition C2 is True
elseif  (V == 4) && (TRIG == 2) && (C(2) == 1) ; V = 1;
% 16) If in State VS AND Trigger ALTCAP occurs THEN transit to ALTS_CAP if condition  [No Condition required] 
elseif  (V == 4) && (TRIG == 4)  ; V = 6;
% 17) If in State VS AND Trigger ALT occurs THEN transit to ALT_HOLD if condition C5 is True
elseif  (V == 4) && (TRIG == 5) && (C(5) == 1) ; V = 5;
% 18) If in State VS AND Trigger SPD occurs THEN transit to SPD_HOLD if condition C3 is True
elseif  (V == 4) && (TRIG == 7) && (C(3) == 1) ; V = 3;
% 19) If in State VS AND Trigger VS occurs THEN transit to PAH if condition  [No Condition required] 
elseif  (V == 4) && (TRIG == 8)  ; V = 2;
% 20) If in State ALT_HOLD AND Trigger APFAIL occurs THEN transit to DIS if condition C2 is True
elseif  (V == 5) && (TRIG == 1) && (C(2) == 1) ; V = 1;
% 21) If in State ALT_HOLD AND Trigger AP occurs THEN transit to DIS if condition C2 is True
elseif  (V == 5) && (TRIG == 2) && (C(2) == 1) ; V = 1;
% 22) If in State ALT_HOLD AND Trigger ALT occurs THEN transit to PAH if condition  [No Condition required] 
elseif  (V == 5) && (TRIG == 5)  ; V = 2;
% 23) If in State ALT_HOLD AND Trigger SPD occurs THEN transit to SPD_HOLD if condition C3 is True
elseif  (V == 5) && (TRIG == 7) && (C(3) == 1) ; V = 3;
% 24) If in State ALT_HOLD AND Trigger VS occurs THEN transit to VS if condition C4 is True
elseif  (V == 5) && (TRIG == 8) && (C(4) == 1) ; V = 4;
% 25) If in State ALTS_CAP AND Trigger APFAIL occurs THEN transit to DIS if condition C2 is True
elseif  (V == 6) && (TRIG == 1) && (C(2) == 1) ; V = 1;
% 26) If in State ALTS_CAP AND Trigger AP occurs THEN transit to DIS if condition C2 is True
elseif  (V == 6) && (TRIG == 2) && (C(2) == 1) ; V = 1;
% 27) If in State ALTS_CAP AND Trigger ALTCPDN occurs THEN transit to ALT_HOLD if condition  [No Condition required] 
elseif  (V == 6) && (TRIG == 3)  ; V = 5;
% 28) If in State ALTS_CAP AND Trigger ALT occurs THEN transit to ALT_HOLD if condition C5 is True
elseif  (V == 6) && (TRIG == 5) && (C(5) == 1) ; V = 5;
end     
%   ================================================
  
% 29) If in State APON AND Trigger APFAIL occurs THEN transit to APOFF if condition  [No Condition required] 
if  (AP == 1) && (TRIG == 1)  ; AP = 2;
% 30) If in State APON AND Trigger AP occurs THEN transit to APOFF if condition  [No Condition required] 
elseif  (AP == 1) && (TRIG == 2)  ; AP = 2;
% 31) If in State APOFF AND Trigger AP occurs THEN transit to APON if condition C1 is True
elseif  (AP == 2) && (TRIG == 2) && (C(1) == 1) ; AP = 1;
end     
%   ================================================
  
% 32) If in State ALTSOFF AND Trigger ALTS occurs THEN transit to ALTSARM if condition  [No Condition required] 
if  (AS == 1) && (TRIG == 6)  ; AS = 2;
% 33) If in State ALTSARM AND Trigger APFAIL occurs THEN transit to ALTSOFF if condition C2 is True
elseif  (AS == 2) && (TRIG == 1) && (C(2) == 1) ; AS = 1;
% 34) If in State ALTSARM AND Trigger AP occurs THEN transit to ALTSOFF if condition C2 is True
elseif  (AS == 2) && (TRIG == 2) && (C(2) == 1) ; AS = 1;
% 35) If in State ALTSARM AND Trigger ALTCAP occurs THEN transit to ALTSCAP if condition  [No Condition required] 
elseif  (AS == 2) && (TRIG == 4)  ; AS = 3;
% 36) If in State ALTSARM AND Trigger ALT occurs THEN transit to ALTSOFF if condition C5 is True
elseif  (AS == 2) && (TRIG == 5) && (C(5) == 1) ; AS = 1;
% 37) If in State ALTSARM AND Trigger ALTS occurs THEN transit to ALTSOFF if condition  [No Condition required] 
elseif  (AS == 2) && (TRIG == 6)  ; AS = 1;
% 38) If in State ALTSCAP AND Trigger APFAIL occurs THEN transit to ALTSOFF if condition C2 is True
elseif  (AS == 3) && (TRIG == 1) && (C(2) == 1) ; AS = 1;
% 39) If in State ALTSCAP AND Trigger AP occurs THEN transit to ALTSOFF if condition C2 is True
elseif  (AS == 3) && (TRIG == 2) && (C(2) == 1) ; AS = 1;
% 40) If in State ALTSCAP AND Trigger ALTCPDN occurs THEN transit to ALTSOFF if condition  [No Condition required] 
elseif  (AS == 3) && (TRIG == 3)  ; AS = 1;
% 41) If in State ALTSCAP AND Trigger ALT occurs THEN transit to ALTSOFF if condition C5 is True
elseif  (AS == 3) && (TRIG == 5) && (C(5) == 1) ; AS = 1;
end     
%   ================================================
  
% ============== Set the outputs ===========
y = zeros(3,1);
y(1) = V;
y(2) = AP;
y(3) = AS;
